simulink subsystem "GUIDANCE_CELESTIALOBJ"  (R2025b)
settings: Solver=VariableStepAuto  StartTime=0.0  StopTime=10.0  RelTol=1e-3
libraries: simulink x3, matrix_library x2, vrlib x2
settings Model: Creator=antoniohernandez-rodiciomateos  LastModifiedBy=antoniohernandez-rodiciomateos

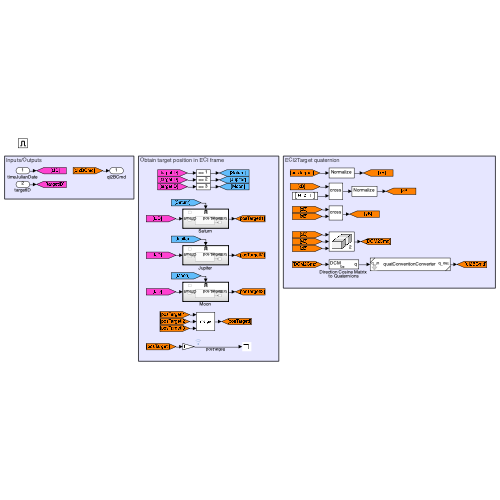
[thumbnail: Simulink's stored preview of the top-level diagram]
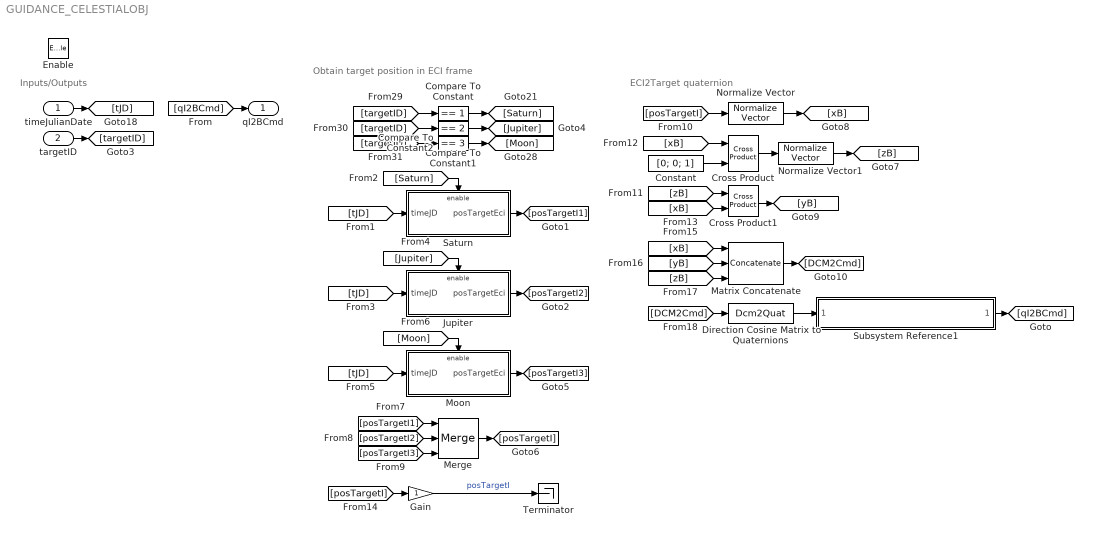
== system GUIDANCE_CELESTIALOBJ ==
  note: Inputs/Outputs
  note: ECI2Target quaternion
  note: Obtain target position in ECI frame
  timeJulianDate : Inport  OutDataTypeStr=double  PortDimensions=[1 1]
  targetID : Inport  Port=2  OutDataTypeStr=double  PortDimensions=[1 1]
  Enable : EnablePort
  Compare To Constant : simulink/Logic and Bit Operations/Compare To Constant  relop===  const=1  OutDataTypeStr=boolean
  Compare To Constant1 : simulink/Logic and Bit Operations/Compare To Constant  relop===  const=2  OutDataTypeStr=boolean
  Compare To Constant2 : simulink/Logic and Bit Operations/Compare To Constant  relop===  const=3  OutDataTypeStr=boolean
  Constant : Constant  Value=[0; 0; 1]
  Cross Product : matrix_library/Cross Product
  Cross Product1 : matrix_library/Cross Product
  Direction Cosine Matrix to Quaternions : Dcm2Quat
  Gain : Gain
  Jupiter : Subsystem
  Matrix Concatenate : Concatenate  NumInputs=3  Mode=Multidimensional array  ConcatenateDimension=2
  Merge : Merge  Inputs=3
  Moon : Subsystem
  Normalize Vector : vrlib/Utilities/Normalize Vector  maxzero=0
  Normalize Vector1 : vrlib/Utilities/Normalize Vector  maxzero=0
  Saturn : Subsystem
  Subsystem Reference1 : Subsystem  ReferencedSubsystem=quatConventionConverter  conversion=q0 to q4
  Terminator : Terminator
  qI2BCmd : Outport
  wires:
  [zB] -> Cross Product1/1
  [posTargetI] -> Gain/1
  targetID/1 -> [targetID]
  Jupiter/1(posTargetEci) -> [posTargetI2]
  Compare To Constant/1 -> [Saturn]
  Gain/1 -> Terminator/1  "posTargetI"
  [xB] -> Cross Product1/2
  [posTargetI3] -> Merge/3
  Matrix Concatenate/1 -> [DCM2Cmd]
  [tJD] -> Saturn/1(timeJD)
  Constant/1 -> Cross Product/2
  Cross Product/1 -> Normalize Vector1/1
  Merge/1 -> [posTargetI]
  Compare To Constant1/1 -> [Jupiter]
  [targetID] -> Compare To Constant/1
  [tJD] -> Jupiter/1(timeJD)
  [posTargetI] -> Normalize Vector/1
  [targetID] -> Compare To Constant1/1
  [posTargetI1] -> Merge/1
  Normalize Vector/1 -> [xB]
  Moon/1(posTargetEci) -> [posTargetI3]
  Cross Product1/1 -> [yB]
  [tJD] -> Moon/1(timeJD)
  timeJulianDate/1 -> [tJD]
  [yB] -> Matrix Concatenate/2
  Subsystem Reference1/1 -> [qI2BCmd]
  [xB] -> Matrix Concatenate/1
  [Saturn] -> Saturn/Enable
  Saturn/1(posTargetEci) -> [posTargetI1]
  [posTargetI2] -> Merge/2
  Normalize Vector1/1 -> [zB]
  [targetID] -> Compare To Constant2/1
  Direction Cosine Matrix to Quaternions/1 -> Subsystem Reference1/1
  [Moon] -> Moon/Enable
  [xB] -> Cross Product/1
  [Jupiter] -> Jupiter/Enable
  [qI2BCmd] -> qI2BCmd/1
  [zB] -> Matrix Concatenate/3
  [DCM2Cmd] -> Direction Cosine Matrix to Quaternions/1
  Compare To Constant2/1 -> [Moon]

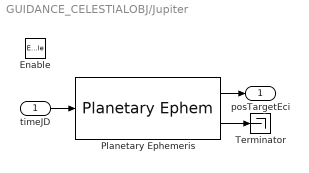
== system GUIDANCE_CELESTIALOBJ/Jupiter ==
  timeJD : Inport  OutDataTypeStr=double  PortDimensions=[1 1]
  Enable : EnablePort
  Planetary Ephemeris : PlanetaryEphem  target=Jupiter
  Terminator : Terminator
  posTargetEci : Outport  OutDataTypeStr=double  PortDimensions=[3 1]
  wires:
  timeJD/1 -> Planetary Ephemeris/1
  Planetary Ephemeris/1 -> posTargetEci/1
  Planetary Ephemeris/2 -> Terminator/1

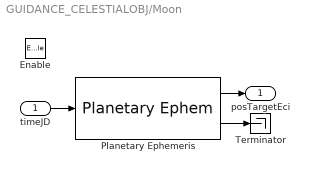
== system GUIDANCE_CELESTIALOBJ/Moon ==
  timeJD : Inport  OutDataTypeStr=double  PortDimensions=[1 1]
  Enable : EnablePort
  Planetary Ephemeris : PlanetaryEphem
  Terminator : Terminator
  posTargetEci : Outport  OutDataTypeStr=double  PortDimensions=[3 1]
  wires:
  timeJD/1 -> Planetary Ephemeris/1
  Planetary Ephemeris/1 -> posTargetEci/1
  Planetary Ephemeris/2 -> Terminator/1

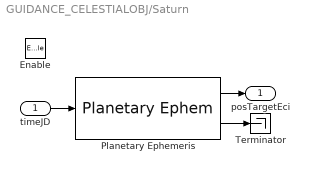
== system GUIDANCE_CELESTIALOBJ/Saturn ==
  timeJD : Inport  OutDataTypeStr=double  PortDimensions=[1 1]
  Enable : EnablePort
  Planetary Ephemeris : PlanetaryEphem  target=Saturn
  Terminator : Terminator
  posTargetEci : Outport  OutDataTypeStr=double  PortDimensions=[3 1]
  wires:
  timeJD/1 -> Planetary Ephemeris/1
  Planetary Ephemeris/1 -> posTargetEci/1
  Planetary Ephemeris/2 -> Terminator/1
